simulink model "ee"  (R2021b)
settings: Solver=VariableStepAuto  StartTime=0.0  StopTime=10.0  RelTol=1e-3
settings Model: Creator=marco  LastModifiedBy=marco

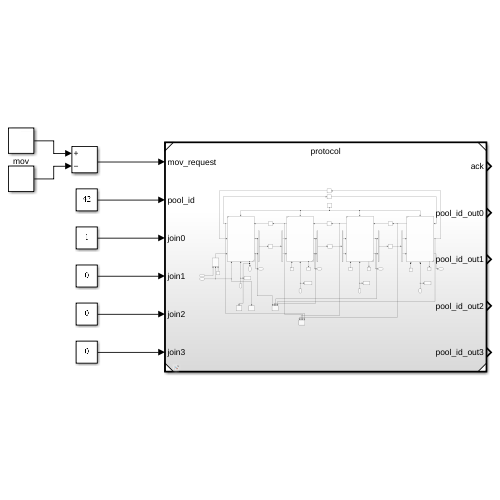
[thumbnail: Simulink's stored preview of the top-level diagram]
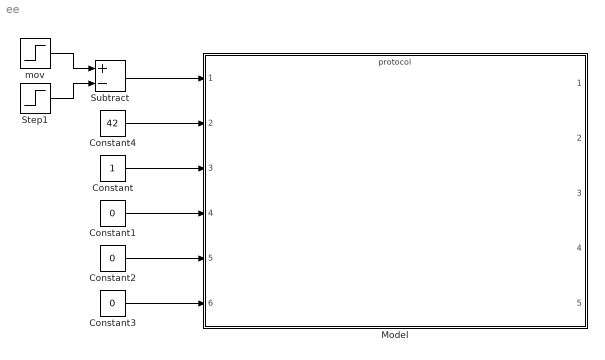
== system ee ==
  Constant : Constant
  Constant1 : Constant  Value=0
  Constant2 : Constant  Value=0
  Constant3 : Constant  Value=0
  Constant4 : Constant  Value=42
  Model : ModelReference  ModelNameDialog=protocol.slx  SimulationMode=Normal  ModelReferenceVersion=1.141
  Step1 : Step  Time=1.2  SampleTime=0.2
  Subtract : Sum  Inputs=+-
  mov : Step  SampleTime=0.2
  wires:
  mov/1 -> Subtract/1
  Step1/1 -> Subtract/2
  Subtract/1 -> Model/1
  Constant/1 -> Model/3
  Constant1/1 -> Model/4
  Constant2/1 -> Model/5
  Constant3/1 -> Model/6
  Constant4/1 -> Model/2
